simulink model "ex8_s"  (R2018b)
settings: Solver=VariableStepAuto  StartTime=0.0  StopTime=10.0  RelTol=1e-3
values from neighbouring files (symbols this model uses):
  A = [-11 -2.5 0;4 0 0;0 0.25 0]    [ex1.m]    (also in ex2.m; ex3.m = sys_s.a; ex4.m = sys_s.A; ex5.m = sys_c.A)
  Astar = sys_z.A    [ex3.m]    (also in ex5.m = sys_star.A; ex6.m = sys_star.A; ex8.m; motore_posizione.m = motore_sysstar.A)
  B = [4 0 0]'    [ex1.m]    (also in ex2.m; ex3.m = sys_s.b; ex4.m = sys_s.B; ex5.m = sys_c.B)
  Bstar = sys_z.B    [ex3.m]    (also in ex5.m = sys_star.B; ex6.m = sys_star.B; ex8.m; motore_posizione.m = motore_sysstar.B)
  C = [0 0 5]    [ex1.m]    (also in ex2.m; ex3.m = sys_s.c; ex4.m = sys_s.C; ex5.m = sys_c.C)
  Cstar = sys_z.C    [ex3.m]    (also in ex5.m = sys_star.C; ex6.m = sys_star.C; ex8.m; motore_posizione.m = motore_sysstar.C)
  H = -acker(A',C',[lam_o lam_o lam_o*10])'    [ex7.m]    (also in ex8.m; motore.m = -acker(A',C',[lam_o lam_o])'; motore_posizione.m = -acker(A',C',[lam_o1 lam_o2 lam_o1])')
  Hstar = -acker(Astar',Cstar',lam_do_star)'    [ex8.m]
  K = -acker(A,B,lam_d)    [ex1.m]    (also in ex2.m; ex3.m = -acker(A,B,lam_ds); ex4.m; ex5.m)
  k_w = k_d/k_F    [ex2.m]    (also in ex3.m; ex4.m; ex5.m; ex6.m)
  k_wstar = k_d/k_Fstar    [ex3.m]    (also in ex8.m; motore_posizione.m = k_d/k_F)
  Kstar = -acker(Astar,Bstar,lam_dz)    [ex3.m]    (also in ex8.m; motore_posizione.m = -acker(Astar,Bstar,lam_dstar))
  T = 0.5/20    (= 0.025)    [ex3.m]    (also in ex5.m = 0.1; ex6.m = 0.2; ex8.m = 0.15; motore_posizione.m = 0.3)
settings Model: Creator=michelemaresca  LastModifiedBy=michelemaresca

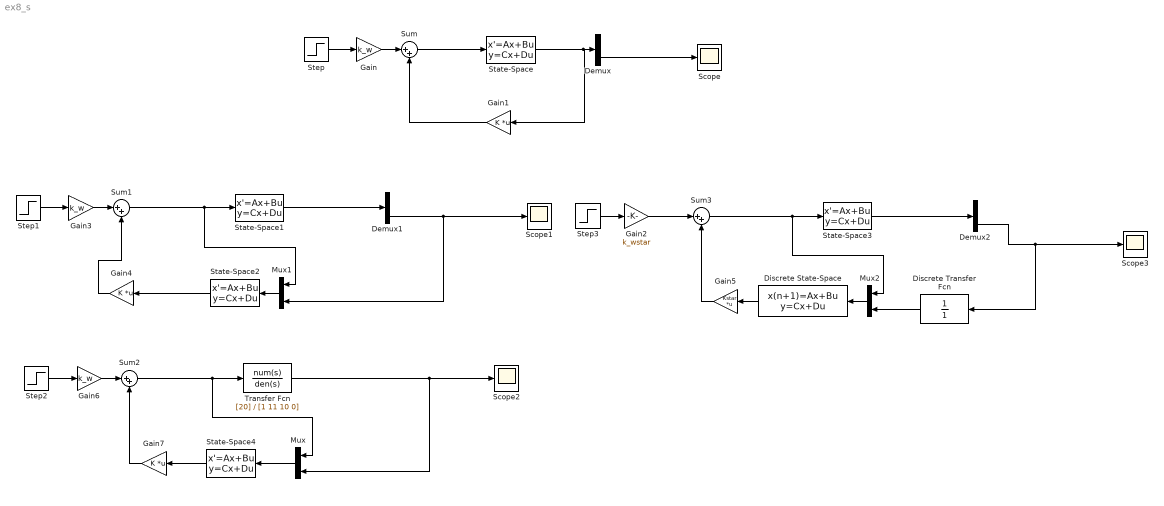
== system ex8_s ==
  Demux : Demux  Outputs=3
  Demux1 : Demux  Outputs=3
  Demux2 : Demux  Outputs=3
  Discrete Transfer Fcn : DiscreteTransferFcn  Denominator=[1]  SampleTime=T
  Discrete State-Space : DiscreteStateSpace  A=Astar+Hstar*Cstar  B=[Bstar -Hstar]  C=eye(3)  D=zeros(3,2)  InitialCondition=[0 0 pi/16]  SampleTime=T
  Gain : Gain  Gain=k_w
  Gain1 : Gain  Gain=K  Multiplication=Matrix(K*u)
  Gain2 : Gain  Gain=k_wstar
  Gain3 : Gain  Gain=k_w
  Gain4 : Gain  Gain=K  Multiplication=Matrix(K*u)
  Gain5 : Gain  Gain=Kstar  Multiplication=Matrix(K*u)
  Gain6 : Gain  Gain=k_w
  Gain7 : Gain  Gain=K  Multiplication=Matrix(K*u)
  Mux : Mux  Inputs=2
  Mux1 : Mux  Inputs=2
  Mux2 : Mux  Inputs=2
  Scope{,1..3} (4 alike) : Scope
  State-Space : StateSpace  A=A  B=B  C=eye(3)  D=zeros(3,1)  InitialCondition=0
  State-Space1 : StateSpace  A=A  B=B  C=eye(3)  D=zeros(3,1)  InitialCondition=0
  State-Space2 : StateSpace  A=A+H*C  B=[B -H]  C=eye(3)  D=zeros(3,2)  InitialCondition=0
  State-Space3 : StateSpace  A=A  B=B  C=eye(3)  D=zeros(3,1)  InitialCondition=0
  State-Space4 : StateSpace  A=A+H*C  B=[B -H]  C=eye(3)  D=zeros(3,2)  InitialCondition=0
  Step : Step  Time=0  SampleTime=0
  Step1 : Step  Time=0  SampleTime=0
  Step2 : Step  Time=0  SampleTime=0
  Step3 : Step  Time=0  SampleTime=T
  Sum{,1..3} (4 alike) : Sum  Inputs=|++
  Transfer Fcn : TransferFcn  Numerator=[20]  Denominator=[1 11 10 0]
  wires:
  Gain3/1 -> Sum1/1
  Step/1 -> Gain/1
  Transfer Fcn/1 -> Mux/2, Scope2/1
  Gain1/1 -> Sum/2
  Gain6/1 -> Sum2/1
  State-Space4/1 -> Gain7/1
  Gain7/1 -> Sum2/2
  Sum/1 -> State-Space/1
  Sum2/1 -> Mux/1, Transfer Fcn/1
  Step2/1 -> Gain6/1
  State-Space/1 -> Demux/1, Gain1/1
  Gain/1 -> Sum/1
  State-Space2/1 -> Gain4/1
  Mux1/1 -> State-Space2/1
  Demux/3 -> Scope/1
  Mux/1 -> State-Space4/1
  Sum1/1 -> Mux1/1, State-Space1/1
  Step1/1 -> Gain3/1
  Gain4/1 -> Sum1/2
  State-Space1/1 -> Demux1/1
  Demux1/3 -> Mux1/2, Scope1/1
  Gain2/1 -> Sum3/1
  State-Space3/1 -> Demux2/1
  Mux2/1 -> Discrete State-Space/1
  Sum3/1 -> Mux2/1, State-Space3/1
  Gain5/1 -> Sum3/2
  Step3/1 -> Gain2/1
  Demux2/3 -> Discrete Transfer Fcn/1, Scope3/1
  Discrete State-Space/1 -> Gain5/1
  Discrete Transfer Fcn/1 -> Mux2/2
